simulink library "lab3lib"  (R2016a)
settings: Solver=ode45  StartTime=0.0  StopTime=10.0  RelTol=1e-3
undefined symbols (not defined in the file or in its folder): robotics
libraries: robotlib x7
settings Model: Creator=andrew  LastModifiedBy=andrew
settings DataIOCC: LimitDataPoints=on
settings DebuggingCC: AllowSymbolicDim=off

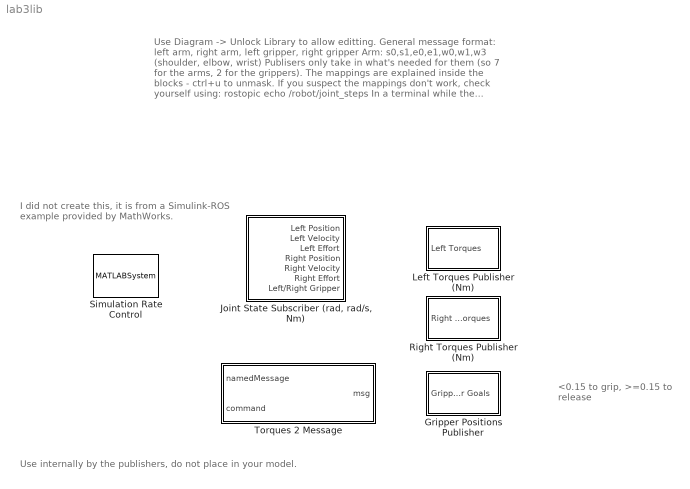
== system lab3lib ==
  note: <0.15 to grip,
      | >=0.15 to release
  note: Use internally by the publishers, do not place in your model.
  note: I did not create this, it is from a
      | Simulink-ROS example provided by
      | MathWorks.
  note: Use Diagram -> Unlock Library to allow editting.
      |
      | General message format: left arm, right arm, left gripper, right gripper
      | Arm: s0,s1,e0,e1,w0,w1,w3 (shoulder, elbow, wrist)
      | Publisers only take in what's needed for them (so 7 for the arms, 2 for
      | the grippers).
      |
      | The mappings are explained inside the blocks - ctrl+u to unmask.
      | If you suspect the mappings don't work, check yourself using:
      | rostopic echo /robot/joint_steps
      | In a terminal while the Baxter simulator or Baxter robot environment is
      | setup and the Robot is running and connected.
  Gripper Positions Publisher : Subsystem  mask(Left Joint Torques){}
      mask help: Outputs the joint position commands to the left and right grippers of either the simulated or physical Baxter robot.
  "Joint State Subscriber (rad, rad/s, Nm)" : Subsystem  mask(Left Joint States){}
      mask help: Gets joints from Baxter.
  Left Torques Publisher (Nm) : Subsystem  mask(Left Joint Torques){}
      mask help: Outputs the joint torque commands to the left arm of either the simulated or physical Baxter robot.
  Right Torques Publisher (Nm) : Subsystem  mask(Left Joint Torques){}
      mask help: Outputs the joint torque commands to the left arm of either the simulated or physical Baxter robot.
  Simulation Rate Control : MATLABSystem  System=ExampleHelperSimulationRateControl  SampleTime=0.02
      mask Type: ExampleHelperSimulationRateControl
      mask Display: disp('Rate Control');
  Torques 2 Message : MATLAB Function  TreatAsAtomicUnit=on

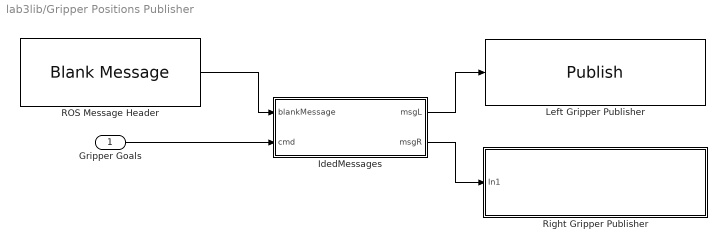
== system lab3lib/Gripper Positions Publisher ==
  Gripper Goals : Inport  PortDimensions=2
  IdedMessages : MATLAB Function  TreatAsAtomicUnit=on
  Left Gripper Publisher : robotlib/Publish  SourceLibraryInfo=This block requires Robotics System Toolbox  topicSource=Select from ROS network  topic=/robot/end_effector/left_gripper/command  messageType=baxter_core_msgs/EndEffectorCommand  messageQueueLength=1
  ROS Message Header : robotlib/Blank Message  SourceLibraryInfo=This block requires Robotics System Toolbox  messageType=baxter_core_msgs/EndEffectorCommand  SampleTime=inf
  Right Gripper Publisher : Subsystem  AncestorBlock=robotlib/Publish  TreatAsAtomicUnit=on  mask(ROS Publish){topicSource=Select from ROS network, topic=/robot/end_effector/right_gripper/command, messageType=baxter_core_msgs/EndEffectorCommand, outputStreamWsVar=, messageQueueLength=1}
      mask prompts: topicSource "robotics:robotslros:blockmask:TopicSourcePrompt"; topic "robotics:robotslros:blockmask:TopicPrompt"; messageType "robotics:robotslros:blockmask:MessageTypePrompt"; outputStreamWsVar "robotics:robotslros:blockmask:PublisherOutputStreamPrompt"; messageQueueLength "robotics:robotslros:blockmask:PublisherMsgQueuePrompt"
      mask help: robotics:robotslros:blockmask:PublisherDescription
      mask init:
      | robotics.slros.internal.block.PublishBlockMask.dispatch('maskInitialize', gcb);
      settings: ModelCloseFcn=robotics.slros.internal.block.PublishBlockMask.dispatch('modelCloseFcn', gcb);
      mask Help: eval('robotics.slros.internal.helpview(''rosPublishBlock'')');
      mask TypeOptions topicSource: Select from ROS network | Specify your own
      mask Callback topicSource: robotics.slros.internal.block.PublishBlockMask.dispatch('topicSourceSelect', gcb);
      mask Callback topic: robotics.slros.internal.block.PublishBlockMask.dispatch('topicEdit', gcb);
      mask TypeOptions outputStreamWsVar: SinkBlock/OutputStreamWsVar
      mask TypeOptions messageQueueLength: SinkBlock/MessageQueueLen
      mask DialogControl id_netAddrLink Prompt: robotics:robotslros:blockmask:ConfigNetworkAddrLinkText
      mask DialogControl id_netAddrLink Callback: robotics.slros.internal.block.PublishBlockMask.dispatch('configureNetworkAddrDlg', gcb);
      mask DialogControl id_topicSelectBtn Prompt: robotics:robotslros:blockmask:SelectPrompt
      mask DialogControl id_topicSelectBtn Callback: robotics.slros.internal.block.PublishBlockMask.dispatch('topicSelect', gcb);
      mask DialogControl id_msgTypeSelectBtn Prompt: robotics:robotslros:blockmask:SelectPrompt
      mask DialogControl id_msgTypeSelectBtn Callback: robotics.slros.internal.block.PublishBlockMask.dispatch('messageTypeSelect', gcb);
      mask Display:
      | color('blue');
      | text(0.2, 0.90, 'ROS', 'horizontalAlignment', 'right');
      | color('black');
      | text(0.5, 0.60, 'Publish', 'horizontalAlignment', 'center');
      | if length(topic) > 20
      |   text(0.95, 0.15, topic, 'horizontalAlignment', 'right');
      | else
      |   text(0.5, 0.15, topic, 'horizontalAlignment', 'center');
      | end
      | port_label('input', 1, 'Msg');
  wires:
  Gripper Goals/1 -> IdedMessages/2(cmd)
  ROS Message Header/1 -> IdedMessages/1(blankMessage)
  IdedMessages/1(msgL) -> Left Gripper Publisher/1
  IdedMessages/2(msgR) -> Right Gripper Publisher/1(In1)

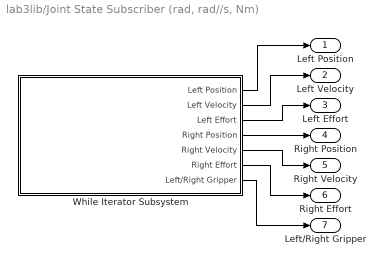
== system lab3lib/Joint State Subscriber (rad, rad//s, Nm) ==
  While Iterator Subsystem : Subsystem  TreatAsAtomicUnit=on
  Left Position : Outport  PortDimensions=7
  Left Velocity : Outport  Port=2  PortDimensions=7
  Left Effort : Outport  Port=3  PortDimensions=7
  Right Position : Outport  Port=4  PortDimensions=7
  Right Velocity : Outport  Port=5  PortDimensions=7
  Right Effort : Outport  Port=6  PortDimensions=7
  Left/Right Gripper : Outport  Port=7  PortDimensions=2
  wires:
  While Iterator Subsystem/4(Right Position) -> Right Position/1
  While Iterator Subsystem/3(Left Effort) -> Left Effort/1
  While Iterator Subsystem/5(Right Velocity) -> Right Velocity/1
  While Iterator Subsystem/2(Left Velocity) -> Left Velocity/1
  While Iterator Subsystem/1(Left Position) -> Left Position/1
  While Iterator Subsystem/6(Right Effort) -> Right Effort/1
  While Iterator Subsystem/7(Left/Right Gripper) -> Left/Right Gripper/1

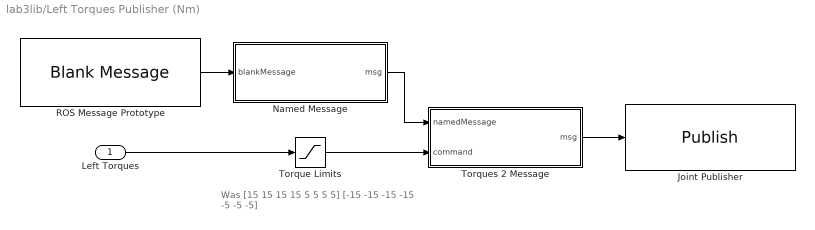
== system lab3lib/Left Torques Publisher (Nm) ==
  note: Was [15 15 15 15 5 5 5 5]
      | [-15 -15 -15 -15 -5 -5 -5]
  Left Torques : Inport  PortDimensions=7
  Joint Publisher : robotlib/Publish  SourceLibraryInfo=This block requires Robotics System Toolbox  topicSource=Select from ROS network  topic=/robot/limb/left/joint_command  messageType=baxter_core_msgs/JointCommand  messageQueueLength=1
  Named Message : MATLAB Function  TreatAsAtomicUnit=on
  ROS Message Prototype : robotlib/Blank Message  SourceLibraryInfo=This block requires Robotics System Toolbox  messageType=baxter_core_msgs/JointCommand  SampleTime=inf
  Torque Limits : Saturate  UpperLimit=[5 5 5 5 5 5 5]  LowerLimit=[-5 -5 -5 -5 -5 -5 -5]
  Torques 2 Message : MATLAB Function  AncestorBlock=lab3lib/Torques 2 Message  TreatAsAtomicUnit=on
  wires:
  Torques 2 Message/1(msg) -> Joint Publisher/1
  Named Message/1(msg) -> Torques 2 Message/1(namedMessage)
  ROS Message Prototype/1 -> Named Message/1(blankMessage)
  Left Torques/1 -> Torque Limits/1
  Torque Limits/1 -> Torques 2 Message/2(command)

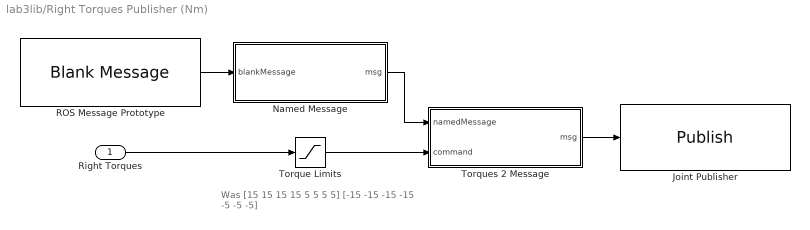
== system lab3lib/Right Torques Publisher (Nm) ==
  note: Was [15 15 15 15 5 5 5 5]
      | [-15 -15 -15 -15 -5 -5 -5]
  Right Torques : Inport  PortDimensions=7
  Joint Publisher : robotlib/Publish  SourceLibraryInfo=This block requires Robotics System Toolbox  topicSource=Select from ROS network  topic=/robot/limb/right/joint_command  messageType=baxter_core_msgs/JointCommand  messageQueueLength=1
  Named Message : MATLAB Function  TreatAsAtomicUnit=on
  ROS Message Prototype : robotlib/Blank Message  SourceLibraryInfo=This block requires Robotics System Toolbox  messageType=baxter_core_msgs/JointCommand  SampleTime=inf
  Torque Limits : Saturate  UpperLimit=[5 5 5 5 5 5 5]  LowerLimit=[-5 -5 -5 -5 -5 -5 -5]
  Torques 2 Message : MATLAB Function  AncestorBlock=lab3lib/Torques 2 Message  TreatAsAtomicUnit=on
  wires:
  Right Torques/1 -> Torque Limits/1
  ROS Message Prototype/1 -> Named Message/1(blankMessage)
  Named Message/1(msg) -> Torques 2 Message/1(namedMessage)
  Torques 2 Message/1(msg) -> Joint Publisher/1
  Torque Limits/1 -> Torques 2 Message/2(command)

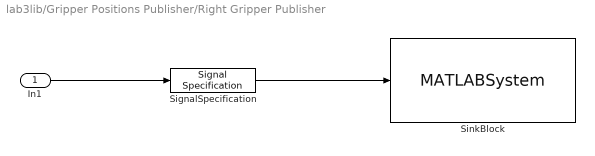
== system lab3lib/Gripper Positions Publisher/Right Gripper Publisher ==
  In1 : Inport  LockScale=on
  SignalSpecification : SignalSpecification  OutDataTypeStr=Bus: SL_Bus_Baxter_PID_baxter_core_msgs_EndEffectorCommand  BusOutputAsStruct=on
      settings: LockScale=on
  SinkBlock : MATLABSystem  InitFcn=robotics.slros.internal.block.PublishBlockMask.dispatch('sysobjInitFcn', gcb);  System=robotics.slros.internal.block.Publisher  ROSTopic=/robot/end_effector/right_gripper/command  ROSMessageType=baxter_core_msgs/EndEffectorCommand  MessageQueueLen=messageQueueLength  SLBusName=SL_Bus_Baxter_PID_baxter_core_msgs_EndEffectorCommand  ModelName=Baxter_PID  BlockId=Pub_Baxter_PID_609  SimulateUsing=Interpreted execution
      mask Type: robotics.slros.internal.block.Publisher
      mask Display:
      | disp('Publisher');
      | port_label('input',1,'busstruct');
  wires:
  In1/1 -> SignalSpecification/1
  SignalSpecification/1 -> SinkBlock/1

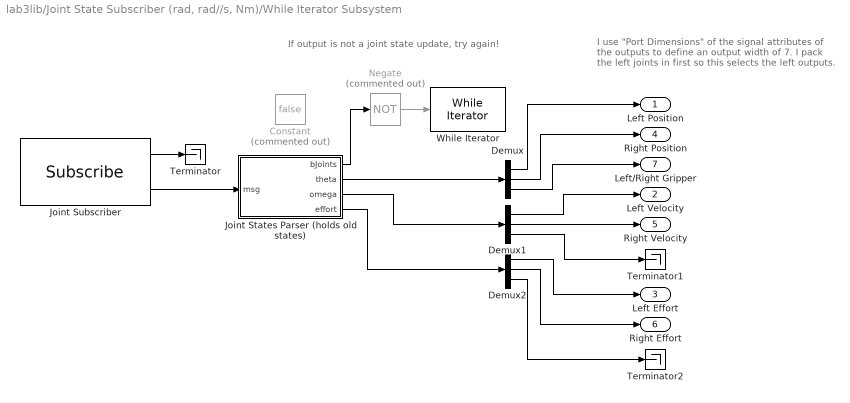
== system lab3lib/Joint State Subscriber (rad, rad//s, Nm)/While Iterator Subsystem ==
  note: If output is not a joint state update, try again!
  note: I use "Port Dimensions" of the signal attributes
      | of the outputs to define an output width of 7.
      | I pack the left joints in first so this selects the left
      | outputs.
  Constant : Constant  Commented=on  Value=false
  Demux : Demux  Outputs=3
  Demux1 : Demux  Outputs=3
  Demux2 : Demux  Outputs=3
  Joint States Parser (holds old states) : MATLAB Function  TreatAsAtomicUnit=on
  Joint Subscriber : robotlib/Subscribe  SourceLibraryInfo=This block requires Robotics System Toolbox  topicSource=Select from ROS network  topic=/robot/joint_states  messageType=sensor_msgs/JointState  sampleTime=-1  messageQueueLength=2
  Negate : Logic  Commented=on  Operator=NOT  AllPortsSameDT=off  OutDataTypeStr=boolean
  Terminator : Terminator
  Terminator1 : Terminator
  Terminator2 : Terminator
  While Iterator : WhileIterator  MaxIters=2  WhileBlockType=do-while
  Left Position : Outport  PortDimensions=7
  Left Velocity : Outport  Port=2  PortDimensions=7
  Left Effort : Outport  Port=3  PortDimensions=7
  Right Position : Outport  Port=4  PortDimensions=7
  Right Velocity : Outport  Port=5  PortDimensions=7
  Right Effort : Outport  Port=6  PortDimensions=7
  Left/Right Gripper : Outport  Port=7  PortDimensions=2
  wires:
  Negate/1 -> While Iterator/1
  Joint Subscriber/1 -> Terminator/1
  Joint Subscriber/2 -> Joint States Parser (holds old states)/1(msg)
  Joint States Parser (holds old states)/1(bJoints) -> Negate/1
  Demux/1 -> Left Position/1
  Demux1/1 -> Left Velocity/1
  Demux2/1 -> Left Effort/1
  Joint States Parser (holds old states)/2(theta) -> Demux/1
  Joint States Parser (holds old states)/3(omega) -> Demux1/1
  Joint States Parser (holds old states)/4(effort) -> Demux2/1
  Demux/2 -> Right Position/1
  Demux/3 -> Left/Right Gripper/1
  Demux1/2 -> Right Velocity/1
  Demux1/3 -> Terminator1/1
  Demux2/2 -> Right Effort/1
  Demux2/3 -> Terminator2/1

== matlab function lab3lib/Gripper Positions Publisher/IdedMessages ==
  data: blankMessage input; msgL output Bus: SL_Bus_Baxter_PID_baxter_core_msgs_EndEffectorCommand; cmd input; msgR output Bus: SL_Bus_Baxter_PID_baxter_core_msgs_EndEffectorCommand
function [msgL,msgR] = namedMsg(blankMessage, cmd)
%#codegen

%% Copy a blank Baxter JointCommand message, fill with data
msg = blankMessage; % Get message prototype from simulink BlankMessage block
msg.Id = uint32(65538);
msg.Args(1:2) = uint8('{}');
msg.Args_SL_Info.CurrentLength = uint32(2);
msg.Sequence = uint32(1);
msg.Sender(1:4) = uint8('host');
msg.Sender_SL_Info.CurrentLength = uint32(4);
msgL = msg; % Copy what's the same
msgR = msg; % Copy what's the same

%% Handle Names field
% What each joint in the command message is - just controlling the grippers
% names={'l_gripper_l_finger_joint'}; %,'r_gripper_l_finger_joint'};
% msg = writeNames(names,msg);
if cmd(1) < 0.015
    msgL.Command(1:4) = uint8('grip');
    msgL.Command_SL_Info.CurrentLength = uint32(4);
else
    msgL.Command(1:7) = uint8('release');
    msgL.Command_SL_Info.CurrentLength = uint32(7);
end

if cmd(2) < 0.015
    msgR.Command(1:4) = uint8('grip');
    msgR.Command_SL_Info.CurrentLength = uint32(4);
else
    msgR.Command(1:7) = uint8('release');
    msgR.Command_SL_Info.CurrentLength = uint32(7);
end

end

== matlab function lab3lib/Left Torques Publisher (Nm)/Named Message ==
  data: blankMessage input; msg output SL_Bus_Baxter_PID_baxter_core_msgs_JointCommand
function msg = namedMsg(blankMessage)
%#codegen

%% Create a blank Baxter JointCommand message, fill with data
msg=blankMessage; % Get message prototype from simulink BlankMessage block

%% Handle Names field
% What each joint in the command message is - just controlling the left arm
% Shoulder 0,1, elbow 0,1, wrist 0,1,2 - moving away from shoulder joint
names={'left_s0','left_s1','left_e0','left_e1','left_w0','left_w1','left_w2'};
msg = writeNames(names,msg);

% Set Mode to torque control
msg.Mode=int32(3); % position mode 1, velocity mode 2, torque mode 3

end

== matlab function lab3lib/Joint State Subscriber (rad, rad//s, Nm)/While Iterator Subsystem/Joint States Parser (holds old states) ==
  data: bJoints output; msg input; theta output; omega output; effort output
function [bJoints,theta,omega,effort] = fcn(msg)
%#codegen

[theta,omega,effort,bJoints] = joint_states(msg,msg.Name_SL_Info.CurrentLength);

== matlab function lab3lib/Torques 2 Message ==
  data: namedMessage input; command input; msg output Bus: SL_Bus_Basic_PID_Tester_baxter_core_msgs_JointCommand
function msg = cmdMsg(namedMessage, command)
%#codegen

%% Create a blank Baxter JointCommand message, fill with data
msg=namedMessage; % Get message prototype from simulink BlankMessage block

%% Handle Command field
msg.Command(1:length(command))=command; %the position you want it to be
msg.Command_SL_Info.CurrentLength=uint32(length(command)); %length of torques

end

== matlab function lab3lib/Right Torques Publisher (Nm)/Named Message ==
  data: blankMessage input; msg output Bus: SL_Bus_Baxter_PID_baxter_core_msgs_JointCommand
function msg = namedMsg(blankMessage)
%#codegen

%% Create a blank Baxter JointCommand message, fill with data
msg=blankMessage; % Get message prototype from simulink BlankMessage block

%% Handle Names field
% What each joint in the command message is - just controlling the right arm
% Shoulder 0,1, elbow 0,1, wrist 0,1,2 - moving away from shoulder joint
names={'right_s0','right_s1','right_e0','right_e1','right_w0','right_w1','right_w2'};
msg = writeNames(names,msg);

% Set Mode to torque control
msg.Mode=int32(3); % position mode 1, velocity mode 2, torque mode 3

end

== matlab function lab3lib/Left Torques Publisher (Nm)/Torques 2 Message ==
  data: namedMessage input; command input; msg output Bus: SL_Bus_Baxter_PID_baxter_core_msgs_JointCommand
function msg = cmdMsg(namedMessage, command)
%#codegen

%% Create a blank Baxter JointCommand message, fill with data
msg=namedMessage; % Get message prototype from simulink BlankMessage block

%% Handle Command field
msg.Command(1:length(command))=command; %the position you want it to be
msg.Command_SL_Info.CurrentLength=uint32(length(command)); %length of torques

end

== matlab function lab3lib/Right Torques Publisher (Nm)/Torques 2 Message ==
  data: namedMessage input; command input; msg output Bus: SL_Bus_Baxter_PID_baxter_core_msgs_JointCommand
function msg = cmdMsg(namedMessage, command)
%#codegen

%% Create a blank Baxter JointCommand message, fill with data
msg=namedMessage; % Get message prototype from simulink BlankMessage block

%% Handle Command field
msg.Command(1:length(command))=command; %the position you want it to be
msg.Command_SL_Info.CurrentLength=uint32(length(command)); %length of torques

end
